simulink model "Pouziti_InterpretedFunction"  (R2020b)
settings: Solver=VariableStepAuto  StartTime=0.0  StopTime=30  RelTol=1e-3
PostLoadFcn:
  | Pouziti_InterpretedFunction_setup;
model workspace (MAT data in the model file):
  b = 2
  g = 9.81
  k = 1000
  m = 1
  x0 = 10
values from neighbouring files (symbols this model uses):
  teleso = rectangle('position',[1 x0 1 1],'FaceColor',[1 0.4 0])    [Pouziti_InterpretedFunction_setup.m]
undefined symbols (not defined in the file or in its folder): posunTelesa
libraries: simulink x1
CloseFcn:
  | clear teleso x0
settings Model: Creator=jirkovsky  LastModifiedBy=jirkovsky
settings DataIOCC: SaveTime=off  ReturnWorkspaceOutputs=off
settings DebuggingCC: ArithmeticOperatorsInVariantConditions=warning
settings SFSimCC: SimUseLocalCustomCode=off  CustomCodeUndefinedFunction=UseInterfaceOnly
settings RTWCC: RTWUseLocalCustomCode=off
settings CodeAppCC: StateflowObjectComments=on

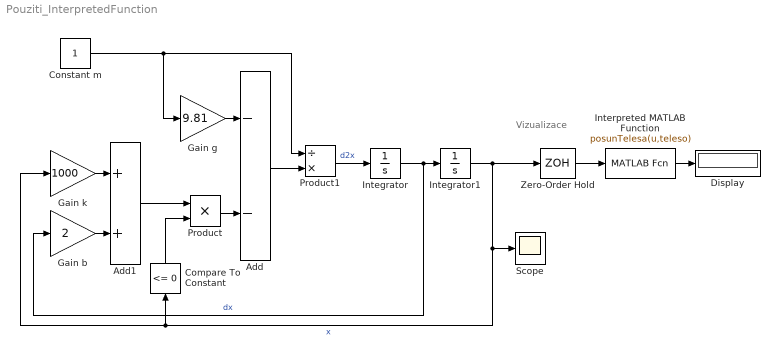
== system Pouziti_InterpretedFunction ==
  note: Vizualizace
  Add : Sum  Inputs=--
  Add1 : Sum
  Compare To Constant : simulink/Logic and Bit Operations/Compare To Constant  relop=<=  const=0  OutDataTypeStr=boolean
  Constant m : Constant
  Display : Display
  Gain b : Gain  Gain=2
  Gain g : Gain  Gain=9.81
  Gain k : Gain  Gain=1000
  Integrator : Integrator
  Integrator1 : Integrator  InitialCondition=x0
  Interpreted MATLAB Function : MATLABFcn  MATLABFcn=posunTelesa(u,teleso)
  Product : Product
  Product1 : Product  Inputs=/*
  Scope : Scope
  Zero-Order Hold : ZeroOrderHold  SampleTime=0.02
  wires:
  Compare To Constant/1 -> Product/2
  Product/1 -> Add/2
  Add1/1 -> Product/1
  Integrator/1 -> Gain b/1, Integrator1/1  "dx"
  Gain g/1 -> Add/1
  Gain k/1 -> Add1/1
  Integrator1/1 -> Zero-Order Hold/1, Scope/1, Compare To Constant/1, Gain k/1  "x"
  Add/1 -> Product1/2
  Product1/1 -> Integrator/1  "d2x"
  Zero-Order Hold/1 -> Interpreted MATLAB Function/1
  Gain b/1 -> Add1/2
  Constant m/1 -> Product1/1, Gain g/1
  Interpreted MATLAB Function/1 -> Display/1
